simulink model "tdc_analog"  (R2020b)
settings: Solver=VariableStepAuto  StartTime=0.0  StopTime=10.0  RelTol=1e-3
values from neighbouring files (symbols this model uses):
  gain_int = 1    [zz_tdc.m]
  vdd = 1.8    [zz_tdc.m]
  vmid_digital = vdd/2    (= 0.9)    [zz_tdc.m]
libraries: simulink x2, simulink_extras x1, dspsigops x1
settings Model: Creator=lydialee  LastModifiedBy=lydialee

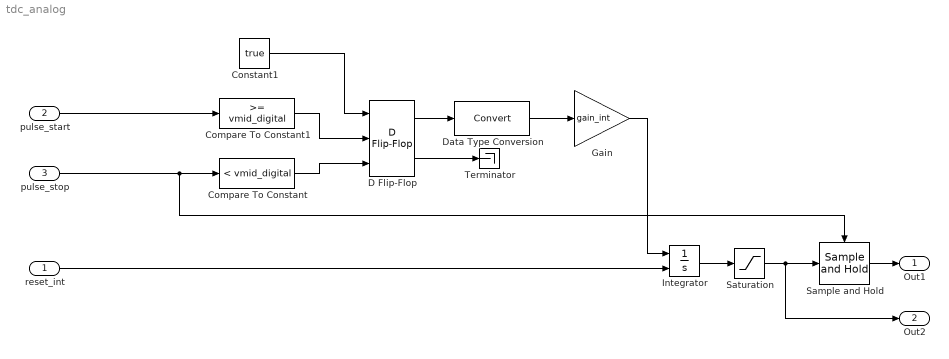
== system tdc_analog ==
  reset_int : Inport
  pulse_start : Inport  Port=2
  pulse_stop : Inport  Port=3
  Compare To Constant : simulink/Logic and Bit Operations/Compare To Constant  relop=<  const=vmid_digital  OutDataTypeStr=boolean
  Compare To Constant1 : simulink/Logic and Bit Operations/Compare To Constant  relop=>=  const=vmid_digital  OutDataTypeStr=boolean
  Constant1 : Constant  Value=true
  D Flip-Flop : simulink_extras/Flip Flops/D Flip-Flop
  Data Type Conversion : DataTypeConversion  OutMin=0  OutMax=1
  Gain : Gain  Gain=gain_int  OutDataTypeStr=Inherit: Same as input
  Integrator : Integrator  ExternalReset=rising
  Sample and Hold : dspsigops/Sample and Hold  trig=Rising edge  initCond=0  latchinput=off
  Saturation : Saturate  UpperLimit=vdd  LowerLimit=0
  Terminator : Terminator
  Out1 : Outport  SignalName=v_TAC
  Out2 : Outport  Port=2  SignalName=v_ramp
  wires:
  Gain/1 -> Integrator/1
  reset_int/1 -> Integrator/2
  Compare To Constant1/1 -> D Flip-Flop/2
  Compare To Constant/1 -> D Flip-Flop/3
  Constant1/1 -> D Flip-Flop/1
  Integrator/1 -> Saturation/1
  pulse_stop/1 -> Sample and Hold/Trigger, Compare To Constant/1
  pulse_start/1 -> Compare To Constant1/1
  Sample and Hold/1 -> Out1/1
  Saturation/1 -> Out2/1, Sample and Hold/1
  D Flip-Flop/1 -> Data Type Conversion/1
  Data Type Conversion/1 -> Gain/1
  D Flip-Flop/2 -> Terminator/1
